simulink model "sysgenFIBONACCI_synth"  (Simulink 6.6)
settings: Solver=VariableStepDiscrete  StartTime=0.0  StopTime=34  MaxStep=1  RelTol=1e-3
libraries: xbsIndex_r4 x16, dspsrcs4 x2, xbsCopyrightNotice_r4 x1
settings Model: Creator=mhirsch  LastModifiedBy=juttu
settings OptimizationCC: InlineInvariantSignals=on
settings DebuggingCC: SignalResolutionControl=TryResolveAllWithWarning  MultiTaskDSMMsg=warning  MultiTaskCondExecSysMsg=none  StrictBusMsg=None
settings RTWCC: IncludeERTFirstTime=on

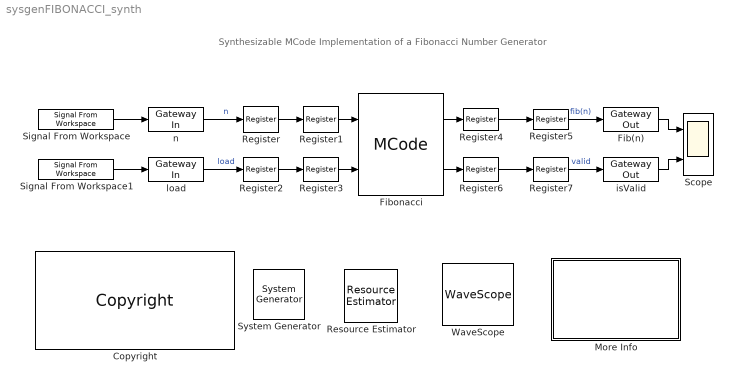
== system sysgenFIBONACCI_synth ==
  note: Synthesizable MCode Implementation
      | of a Fibonacci Number Generator
  " System Generator" : xbsIndex_r4/ System Generator  Tag=genX  SystemSampleTime=-1  xilinxfamily=Virtex4  part=xc4vsx35  speed=-10  package=ff668  synthesis_tool=XST  clock_wrapper=Clock Enables  directory=./netlist  testbench=off  simulink_period=1  sysclk_period=5  dcm_input_clock_period=100  incr_netlist=off  trim_vbits=Everywhere in SubSystem  dbl_ovrd=According to Block Masks  core_generation=According to Block Masks  run_coregen=off  deprecated_control=off  eval_field=0  block_type=sysgen
      settings: block_version=9.2.00
  Copyright : xbsCopyrightNotice_r4/Copyright  block_type=copyright
      settings: block_version=10.1.00
      settings: infoedit=|
      | Copyright(C) 2008 by  Xilinx, Inc. All rights reserved.<br>
      | <br>
      | This file contains proprietary, confidential information of Xilinx, Inc., is distributed under license
      | from Xilinx, Inc., and may be used, copied and/or disclosed only pursuant to the terms of a valid license
      | agreement with Xilinx, Inc. Xilinx hereby grants you a license to use this file solely for design,
      | simulation, implementation and creation of design files limited to Xilinx devices or technologies. Use
      | with non-Xilinx devices or technologies is expressly prohibited and immediately terminates your license
      | unless covered by a separate agreement.<br>
      | <br>
      | Xilinx is providing this design, code, or information "as-is" solely for use in developing programs and
      | solutions for Xilinx devices, with no obligation on the part of Xilinx to provide support. By providing
      | this design, code, or information as one possible implementation of this feature, application or standard,
      | Xilinx is making no representation that this implementation is free from any claims of infringement. You
      | are responsible for obtaining any rights you may require for your implementation. Xilinx expressly disclaims
      | any warranty whatsoever with respect to the adequacy of the implementation, including but not limited to any
      | warranties or representations that this implementation is free from claims of infringement, implied warranties
      | of merchantability or fitness for a particular purpose.<br>
      | <br>
      | Xilinx products are not intended for use in life support appliances, devices, or systems. Use in such
      | applications is expressly prohibited.<br>
      | <br>
      | Any modifications that are made to the Source Code are done at the user's sole risk and will be unsupported.<br>
      | <br>
      | This copyright and support notice must be retained as part of this text at all times.
      | (c) Copyright 1995-2008 Xilinx, Inc. All rights reserved.
  Fib(n) : xbsIndex_r4/Gateway Out  hdl_port=on  timing_constraint=None  locs_specified=off  LOCs={}  block_type=gatewayout
      settings: infoedit="Gateway out block.  Converts Xilinx fixed point inputs into ouputs of type Simulink integer, double, or fixed point.<P><P>Hardware notes:  In hardware these blocks become top level output ports or are discarded, depending on how they are configured."  block_version=VER_STRING_GOES_HERE
  Fibonacci : xbsIndex_r4/MCode  mfname=sysgenFibonacci  explicit_period=off  period=1  dbl_ovrd=off  enable_stdout=off  enable_debug=off  suppress_output=1  defparams={}  hide_port_list={}  block_type=mcode
      settings: block_version=8.1
  More Info : Subsystem
      mask Display: disp('Double click\n for\n more information.')
  Register{,1,4..7} (6 alike) : xbsIndex_r4/Register  init=0  rst=off  en=off  dbl_ovrd=off  block_type=register
      settings: block_version=VER_STRING_GOES_HERE
  Register2 : xbsIndex_r4/Register  init=1  rst=off  en=off  dbl_ovrd=off  block_type=register
      settings: block_version=VER_STRING_GOES_HERE
  Register3 : xbsIndex_r4/Register  init=1  rst=off  en=off  dbl_ovrd=off  block_type=register
      settings: block_version=VER_STRING_GOES_HERE
  Resource Estimator : xbsIndex_r4/Resource Estimator  Tag=resEstTag  Slices=109  FFs=144  BRAMs=0  LUTs=78  IOBs=0  EBMs=0  TBUFs=0  xl_use_estimator_area=off  est_options=Post Map  block_type=resource_estimator
      settings: AttributesFormatString=Resource\nEstimator  block_version=9.2.00
  Scope : Scope  NumInputPorts=2
      settings: YMin=-5~-5  YMax=5~5
  Signal From Workspace : dspsrcs4/Signal From Workspace  SystemSampleTime=-1  X=[5 zeros(1,9) 1 zeros(1,9) 8]  Ts=1  nsamps=1  OutputAfterFinalValue=Setting to zero  ignoreOrWarnInputAndFrameLengths=off
  Signal From Workspace1 : dspsrcs4/Signal From Workspace  SystemSampleTime=-1  X=[1 zeros(1,9) 1 zeros(1,9) 1 zeros(1,9) 1]  Ts=1  nsamps=1  OutputAfterFinalValue=Setting to zero  ignoreOrWarnInputAndFrameLengths=off
  WaveScope : xbsIndex_r4/WaveScope  block_type=wavescope
      settings: block_version=9.2.00
  isValid : xbsIndex_r4/Gateway Out  hdl_port=on  timing_constraint=None  locs_specified=off  LOCs={}  block_type=gatewayout
      settings: infoedit="Gateway out block.  Converts Xilinx fixed point inputs into ouputs of type Simulink integer, double, or fixed point.<P><P>Hardware notes:  In hardware these blocks become top level output ports or are discarded, depending on how they are configured."  block_version=VER_STRING_GOES_HERE
  load : xbsIndex_r4/Gateway In  arith_type=Boolean  n_bits=8  bin_pt=0  quantization="Round  (unbiased: +/- Inf)"  overflow=Saturate  period=1  dbl_ovrd=off  timing_constraint=None  locs_specified=off  LOCs={}  block_type=gatewayin
      settings: infoedit="Gateway in block.  Converts inputs of type Simulink integer, double and fixed point to  Xilinx fixed point type.<P><P>Hardware notes:  In hardware these blocks become top level input ports."  block_version=VER_STRING_GOES_HERE
  n : xbsIndex_r4/Gateway In  arith_type=Unsigned  n_bits=8  bin_pt=0  quantization="Round  (unbiased: +/- Inf)"  overflow=Saturate  period=1  dbl_ovrd=off  timing_constraint=None  locs_specified=off  LOCs={}  block_type=gatewayin
      settings: infoedit="Gateway in block.  Converts inputs of type Simulink integer, double and fixed point to  Xilinx fixed point type.<P><P>Hardware notes:  In hardware these blocks become top level input ports."  block_version=VER_STRING_GOES_HERE
  wires:
  Signal From Workspace1/1 -> load/1
  Signal From Workspace/1 -> n/1
  load/1 -> Register2/1  "load"
  Fibonacci/2 -> Register6/1
  n/1 -> Register/1  "n"
  Fibonacci/1 -> Register4/1
  Register6/1 -> Register7/1
  Register7/1 -> isValid/1  "valid"
  Register4/1 -> Register5/1
  Register5/1 -> Fib(n)/1  "fib(n)"
  Register/1 -> Register1/1
  Register1/1 -> Fibonacci/1
  Register3/1 -> Fibonacci/2
  Register2/1 -> Register3/1
  Fib(n)/1 -> Scope/1
  isValid/1 -> Scope/2

== system sysgenFIBONACCI_synth/More Info ==
  note: This design implements a Fibonacci number generator in an MCode block.  That is, given a non-negative integer n, it computes the
      | recursively defined sequence x_0 = 1, x_1 = 1, ... , n_n = x_{n-2} + x_{n-1}.
      |
      | This design should be compared to sysgenFibonacciLogic which implements the same computation in a more hardware-centric way.
      | The m-code implementing the MCode block is written so as to be as close as possible to the logic in sysgenFibCores.  It is instructional
      | to look at the m-code to learn how to implement an efficient MCode block.
      |
      | The two designs are functionally equivalent, and use the same amount of FPGA resources.
      |
      | For correctness of the design in practice, all the I/O gateways should be double buffered.  This design does not do this for simplicity.
      | The comparison of the logic design and the MCode design is simpler without the double buffering.
  note: MCode-Based Fibonacci Sequence
